simulink model "gm_spectrum_analyser"  (R2020a)
settings: Solver=VariableStepAuto  StartTime=0.0  StopTime=100000/256e6  RelTol=1e-3
InitFcn:
  | fs = 256e6;
undefined symbols (not defined in the file or in its folder): designMultirateFIR
libraries: hdlsllib x81, simulink x50, dspmlti4 x6, dsphdlxfrm x5, hdlmdlgenlib x4, dspswit3 x4, dspsigops x2, dspsigattribs x2
(part 2 of 5)

== system gm_spectrum_analyser/Stimulus and Channel/Channel/RF-DAC ==
  Valid : Inport
  Data : Inport  Port=2
  Interpolation Filter : Subsystem  mask{interp=4x}
      mask prompts: interp "Interpolation Factor:"
      mask init:
      | fir0 = dsp.FIRInterpolator('InterpolationFactor', 2,...
      |                            'CoefficientsDataType', 'Custom',...
      |                            'CustomCoefficientsDataType', numerictype([], 16, 14),...
      |                            'FullPrecisionOverride', false,...
      |                            'OutputDataType', 'Custom',...
      |                            'CustomOutputDataType', numerictype([], 16, 15),...
      |                            'Numerator', [-6, 0 54, 0, -254, 0, 1230, 2048, 1230, 0, -254, 0, 54, 0, -6]/(2048));
      | fir1 = dsp.FIRInterpolator('InterpolationFactor', 2,...
      |                            'CoefficientsDataType', 'Custom',...
      |                            'CustomCoefficientsDataType', numerictype([], 16, 14),...
      |                            'FullPrecisionOverride', false,...
      |                            'OutputDataType', 'Custom',...
      |                            'CustomOutputDataType', numerictype([], 16, 15),...
      |                            'Numerator', [-12, 0, 84, 0, -337, 0, 1008, 0, -2693, 0, 10142, 16384, 10142, 0, -2693, 0, 1008, 0, -337, 0, 84, 0 ,-12]/(16384));
      | fir2 = dsp.FIRInterpolator('InterpolationFactor', 2,...
      |                            'CoefficientsDataType', 'Custom',...
      |                            'CustomCoefficientsDataType', numerictype([], 16, 14),...
      |                            'FullPrecisionOverride', false,...
      |                            'OutputDataType', 'Custom',...
      |                            'CustomOutputDataType', numerictype([], 16, 15),...
      |                            'Numerator', [5, 0, -17, 0, 44, 0, -96, 0, 187, 0, -335, 0, 565, 0, -906, 0, 1401, 0, -2112, 0, 3145, 0, -4723, 0, 7415, 0, -13331, 0, 41526, 65536, 41526, 0, -13331, 0, 7415, 0, -4723, 0, 3145, 0, -2112, 0, 1401, 0, -906, 0, 565, 0, -335, 0, 187, 0, -96, 0, 44, 0, -17, 0, 5]/(65536));
      | switch get_param(gcb, 'interp')
      |     case '1x'
      |         if ~strcmp(get_param([gcb, '/FIR 0'], 'Commented'), 'through')
      |             set_param([gcb, '/FIR 0'],'Commented','through');
      |         end
      |         
      |         if ~strcmp(get_param([gcb, '/FIR 1'], 'Commented'), 'through')
      |             set_param([gcb, '/FIR 1'],'Commented','through');
      |         end
      |         
      |         if ~strcmp(get_param([gcb, '/FIR 2'], 'Commented'), 'through')
      |             set_param([gcb, '/FIR 2'],'Commented','through');
      |         end
      |             
      |     case '2x'
      |         if ~strcmp(get_param([gcb, '/FIR 0'], 'Commented'), 'through')
      |             set_param([gcb, '/FIR 0'],'Commented','through');
      |         end
      |         
      |         if ~strcmp(get_param([gcb, '/FIR 1'], 'Commented'), 'through')
      |             set_param([gcb, '/FIR 1'],'Commented','through');
      |         end
      |         
      |         if ~strcmp(get_param([gcb, '/FIR 2'], 'Commented'), 'off')
      |             set_param([gcb, '/FIR 2'],'Commented','off');
      |         end
      | 
      |     case '4x'
      |         if ~strcmp(get_param([gcb, '/FIR 0'], 'Commented'), 'through')
      |             set_param([gcb, '/FIR 0'],'Commented','through');
      |         end
      |         
      |         if ~strcmp(get_param([gcb, '/FIR 1'], 'Commented'), 'off')
      |             set_param([gcb, '/FIR 1'],'Commented','off');
      |         end
      |         
      |         if ~strcmp(get_param([gcb, '/FIR 2'], 'Commented'), 'off')
      |             set_param([gcb, '/FIR 2'],'Commented','off');
      |         end
      |         
      |     case '8x'
      |         if ~strcmp(get_param([gcb, '/FIR 0'], 'Commented'), 'off')
      |             set_param([gcb, '/FIR 0'],'Commented','off');
      |         end
      |         
      |         if ~strcmp(get_param([gcb, '/FIR 1'], 'Commented'), 'off')
      |             set_param([gcb, '/FIR 1'],'Commented','off');
      |         end
      |         
      |         if ~strcmp(get_param([gcb, '/FIR 2'], 'Commented'), 'off')
      |             set_param([gcb, '/FIR 2'],'Commented','off');
      |         end
      | 
      | end
      mask TypeOptions interp: 1x | 2x | 4x | 8x
      mask DialogControl DescGroupVar Prompt: RF-DAC Interpolation Filter
      mask DialogControl DescTextVar Prompt: This block simulates the RF-DAC interpolation stage using the same coefficients stored in the interpolation filters.
      mask DialogControl ParameterGroupVar Prompt: Main
  NCO and Mixer : Subsystem
  RF-DAC : Subsystem
  SSR Converter RF-DAC : Subsystem
  Data Out : Outport  VectorParamsAs1DForOutWhenUnconnected=off
  wires:
  RF-DAC/1(Data Out) -> Data Out/1
  NCO and Mixer/1(Data Out) -> RF-DAC/1(Data In)
  Interpolation Filter/1(Data Out) -> NCO and Mixer/1(Data In)
  Data/1 -> SSR Converter RF-DAC/2(Data)
  Valid/1 -> SSR Converter RF-DAC/1(Valid)
  SSR Converter RF-DAC/1(Data Out) -> Interpolation Filter/1(Data In)

== system gm_spectrum_analyser/Stimulus and Channel/Transmitter/Transmitter ==
  Enable : Inport
  Value : Inport  Port=2
  Bit Concat : hdlsllib/Logic and Bit Operations/Bit Concat  numInputs=2
  Bit Slice : hdlsllib/Logic and Bit Operations/Bit Slice  lidx=15  ridx=0
      settings: SourceProductBaseCode=SL
  Bit Slice1 : hdlsllib/Logic and Bit Operations/Bit Slice  lidx=31  ridx=16
      settings: SourceProductBaseCode=SL
  Complex to Real-Imag : ComplexToRealImag
  Constant : Constant  OutDataTypeStr=boolean  SampleTime=-1
  Constant2 : Constant  Value=[0, 0, 0, 0]'  VectorParams1D=off  OutDataTypeStr=fixdt(1,16,15)  SampleTime=-1
  Data Type Conversion : DataTypeConversion  OutDataTypeStr=fixdt(1,16,15)  ConvertRealWorld=Stored Integer (SI)
  Data Type Conversion1 : DataTypeConversion  OutDataTypeStr=fixdt(1,16,15)  ConvertRealWorld=Stored Integer (SI)
  Matrix Concatenate : Concatenate  NumInputs=4  Mode=Multidimensional array
  Multiport Switch : MultiPortSwitch  DataPortOrder=Zero-based contiguous  Inputs=2  zeroidx=on
  Real-Imag to Complex : RealImagToComplex
  Real-Imag to Complex1 : RealImagToComplex
  Vector to SSR Low : Subsystem  mask{N=4, hN=4}
      mask prompts: N "Samples per clock cycle:"
      mask init:
      | if ~isequal(get_param(gcb, 'N'), get_param(gcb, 'hN'))
      |     % Delete all blocks except input and output ports
      |     delete_block(setxor(setdiff(...
      |         find_system(gcb,'LookUnderMasks','on'),...
      |         {[gcb, '/Vector'], [gcb, '/SSR']}), gcb));
      | 
      |     % Delete all wires
      |     delete_line(find_system(gcb, 'FindAll', 'on', 'LookUnderMasks',...
      |         'on', 'SearchDepth', 3, 'Type', 'line', 'Connected', 'off'));
      | 
      |     % Add the bit concatenation block
      |     add_block('hdlsllib/Logic and Bit Operations/Bit Concat',...
      |         [gcb, '/Bit Concat'],...
      |         'Position', [155 55 205 330]);
      |     set_param([gcb, '/Bit Concat'], 'numInputs', num2str(N));
      | 
      |     % Add wire to output
      |     add_line(gcb, 'Bit Concat/1', 'SSR/1');
      | 
      |     % Add selector blocks and connect wires
      |     for i = 0:N-1
      |         add_block('simulink/Signal Routing/Selector',...
      |             [gcb, '/Selector', num2str(i)],...
      |             'Position', [0 82+i*90 45 128+i*90]);
      |         set_param([gcb, '/Selector', num2str(i)], 'InputPortWidth', num2str(N));
      |         set_param([gcb, '/Selector', num2str(i)], 'IndexParamArray', {num2str(N-i)});
      |         add_line(gcb, 'Vector/1', ['Selector', num2str(i), '/1'],...
      |             'autorouting', 'on');
      |         add_line(gcb, ['Selector', num2str(i), '/1'],...
      |             ['Bit Concat/', num2str(i+1)],...
      |             'autorouting', 'on');
      |     end
      |     
      |     % Set the hidden attribute to prevent unnecessary changes in
      |     % architecture while generating HDL Code.
      |     set_param(gcb, 'hN', get_param(gcb, 'N'));
      | end
      mask DialogControl DescGroupVar Prompt: Vector to SSR
      mask DialogControl DescTextVar Prompt: Convert a vector of inputs into SSR format.
  Valid : Outport
  Data : Outport  Port=2
  wires:
  Complex to Real-Imag/2 -> Bit Concat/1
  Vector to SSR Low/1(SSR) -> Data/1
  Complex to Real-Imag/1 -> Bit Concat/2
  Bit Concat/1 -> Vector to SSR Low/1(Vector)
  Multiport Switch/1 -> Complex to Real-Imag/1
  Constant2/1 -> Real-Imag to Complex/2, Real-Imag to Complex/1
  Real-Imag to Complex/1 -> Multiport Switch/2
  Enable/1 -> Multiport Switch/1
  Value/1 -> Bit Slice1/1, Bit Slice/1
  Data Type Conversion/1 -> Real-Imag to Complex1/1
  Bit Slice/1 -> Data Type Conversion/1
  Bit Slice1/1 -> Data Type Conversion1/1
  Data Type Conversion1/1 -> Real-Imag to Complex1/2
  Constant/1 -> Valid/1
  Real-Imag to Complex1/1 -> Matrix Concatenate/4, Matrix Concatenate/3, Matrix Concatenate/2, Matrix Concatenate/1
  Matrix Concatenate/1 -> Multiport Switch/3

== system gm_spectrum_analyser/DDR Memory/AXI Read Interface Response Model/DDR/Enabled Subsystem ==
  rd_addr : Inport
  rd_len : Inport  Port=2
  rd_avalid : Inport  Port=3
  Enable : EnablePort
  Compare To Constant : simulink/Logic and Bit Operations/Compare To Constant  relop===  const=1  OutDataTypeStr=boolean
  Constant : Constant  Value=4  SampleTime=-1
  Constant1 : Constant  OutDataTypeStr=boolean  SampleTime=-1
  Delay : Delay  DelayLength=1
  Direct Lookup Table (n-D) : LookupNDDirect  NumberOfTableDimensions=1  Table=DDR_DATA  DiagnosticForOutOfRangeInput=Error
  HDL Counter : hdlsllib/Sources/HDL Counter  CountType=Count limited  CountInit=0  CountStep=1  CountMax=2^16-1  CountFromType=Specify  CountFrom=0  CountResetPort=on  CountLoadPort=off  CountEnbPort=on  CountDirPort=off  CountDataType=Unsigned  CountWordLen=16  CountFracLen=0  CountSampTime=1
  MATLAB Function : MATLAB Function  TreatAsAtomicUnit=on
  Product : Product  Inputs=*/
  Sum : Sum  Inputs=|++  OutDataTypeStr=uint32
  Sum1 : Sum  Inputs=|+-
  latch : Subsystem
  rd_data : Outport  VectorParamsAs1DForOutWhenUnconnected=off
  rd_aready : Outport  Port=2  VectorParamsAs1DForOutWhenUnconnected=off
  rd_dvalid : Outport  Port=3  VectorParamsAs1DForOutWhenUnconnected=off
  wires:
  Constant1/1 -> rd_aready/1
  Delay/1 -> MATLAB Function/2(rst)
  Constant/1 -> Product/2
  Product/1 -> Sum/1
  latch/1(q) -> Product/1
  MATLAB Function/1(start_counter) -> HDL Counter/2, rd_dvalid/1
  rd_avalid/1 -> MATLAB Function/1(rd_avalid), latch/1(e)
  rd_len/1 -> Sum1/1
  rd_addr/1 -> latch/2(d)
  Compare To Constant/1 -> HDL Counter/1, Delay/1
  Sum/1 -> Direct Lookup Table (n-D)/1
  Sum1/1 -> Compare To Constant/1
  HDL Counter/1 -> Sum/2, Sum1/2  "addr_inc"
  Direct Lookup Table (n-D)/1 -> rd_data/1

== system gm_spectrum_analyser/DDR Memory/AXI Write Interface Response Model/Serial to FFT Frame/Enabled Subsystem2 ==
  Data In : Inport
  Enable : EnablePort
  Buffer : Buffer  N=N  OutputFrames=off
  Data Out : Outport
  wires:
  Data In/1 -> Buffer/1
  Buffer/1 -> Data Out/1

== system gm_spectrum_analyser/Spectrum Analyser/Spectrum Analyser/Direct Memory Access/Direct Memory Access ==
  Length : Inport  OutDataTypeStr=uint32  PortDimensions=1  SampleTime=3.90625e-09
  Count : Inport  Port=2  OutDataTypeStr=uint32  PortDimensions=1  SampleTime=3.90625e-09
  Buffer Address 1 : Inport  Port=3  OutDataTypeStr=uint32  PortDimensions=1  SampleTime=3.90625e-09
  Buffer Address 2 : Inport  Port=4  OutDataTypeStr=uint32  PortDimensions=1  SampleTime=3.90625e-09
  Buffer Address 3 : Inport  Port=5  OutDataTypeStr=uint32  PortDimensions=1  SampleTime=3.90625e-09
  Enable DMA : Inport  Port=6  OutDataTypeStr=uint32  PortDimensions=1  SampleTime=3.90625e-09
  Valid In : Inport  Port=7  OutDataTypeStr=boolean  PortDimensions=1  SampleTime=3.90625e-09
  Data In : Inport  Port=8  OutDataTypeStr=uint32  PortDimensions=1  SampleTime=3.90625e-09
  Start In : Inport  Port=9  OutDataTypeStr=boolean  PortDimensions=1  SampleTime=3.90625e-09
  End In : Inport  Port=10  OutDataTypeStr=boolean  PortDimensions=1  SampleTime=3.90625e-09
  wr_ready : Inport  Port=11  SampleTime=3.90625e-09
  DDR Communication : Subsystem
  wr_data : Outport
  wr_m2s : Outport  Port=2
  Buffer Pointer : Outport  Port=3
  DMA Status : Outport  Port=4
  wires:
  DDR Communication/1(Buffer Pointer) -> Buffer Pointer/1
  DDR Communication/2(wr_data) -> wr_data/1
  DDR Communication/3(wr_m2s) -> wr_m2s/1
  DDR Communication/4(DMA Status) -> DMA Status/1
  Length/1 -> DDR Communication/1(Length)
  Count/1 -> DDR Communication/2(Count)
  Buffer Address 1/1 -> DDR Communication/3(Buffer Address 1)
  Buffer Address 2/1 -> DDR Communication/4(Buffer Address 2)
  Buffer Address 3/1 -> DDR Communication/5(Buffer Address 3)
  Enable DMA/1 -> DDR Communication/6(Enable)
  Valid In/1 -> DDR Communication/7(Valid Out)
  Data In/1 -> DDR Communication/8(Data Out)
  Start In/1 -> DDR Communication/9(Start In)
  End In/1 -> DDR Communication/10(End In)
  wr_ready/1 -> DDR Communication/11(wr_ready)

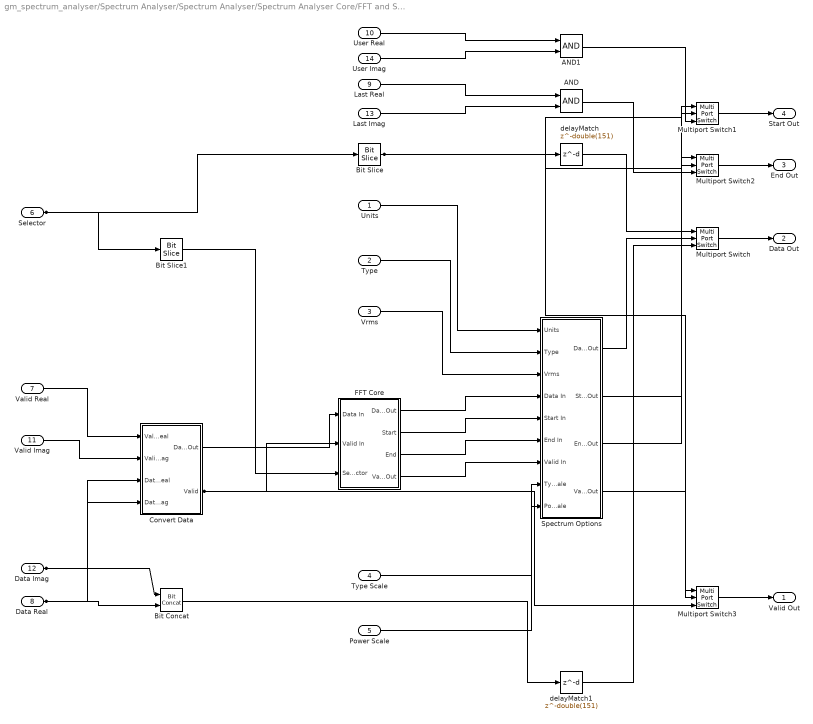
== system gm_spectrum_analyser/Spectrum Analyser/Spectrum Analyser/Spectrum Analyser Core/FFT and Spectrum Processing ==
  Units : Inport  OutDataTypeStr=uint32  SampleTime=3.90625e-09
  Type : Inport  Port=2  OutDataTypeStr=uint32  SampleTime=3.90625e-09
  Vrms : Inport  Port=3  OutDataTypeStr=uint32  SampleTime=3.90625e-09
  Type Scale : Inport  Port=4  OutDataTypeStr=uint32  SampleTime=3.90625e-09
  Power Scale : Inport  Port=5  OutDataTypeStr=uint32  SampleTime=3.90625e-09
  Selector : Inport  Port=6  OutDataTypeStr=uint32  SampleTime=3.90625e-09
  Valid Real : Inport  Port=7  OutDataTypeStr=boolean  SampleTime=3.90625e-09
  Data Real : Inport  Port=8  OutDataTypeStr=uint16  SampleTime=3.90625e-09
  Last Real : Inport  Port=9  OutDataTypeStr=boolean  SampleTime=3.90625e-09
  User Real : Inport  Port=10  OutDataTypeStr=boolean  SampleTime=3.90625e-09
  Valid Imag : Inport  Port=11  OutDataTypeStr=boolean  SampleTime=3.90625e-09
  Data Imag : Inport  Port=12  OutDataTypeStr=uint16  SampleTime=3.90625e-09
  Last Imag : Inport  Port=13  OutDataTypeStr=boolean  SampleTime=3.90625e-09
  User Imag : Inport  Port=14  OutDataTypeStr=boolean  SampleTime=3.90625e-09
  AND : Logic  AllPortsSameDT=off  OutDataTypeStr=boolean  SampleTime=3.90625e-09
  AND1 : Logic  AllPortsSameDT=off  OutDataTypeStr=boolean  SampleTime=3.90625e-09
  Bit Concat : hdlsllib/Logic and Bit Operations/Bit Concat  numInputs=2
  Bit Slice : hdlsllib/Logic and Bit Operations/Bit Slice  lidx=double(8)  ridx=double(8)
      settings: SourceProductBaseCode=SL
  Bit Slice1 : hdlsllib/Logic and Bit Operations/Bit Slice  lidx=double(7)  ridx=double(0)
      settings: SourceProductBaseCode=SL
  Convert Data : Subsystem
  FFT Core : Subsystem
  Multiport Switch : MultiPortSwitch  DataPortOrder=Zero-based contiguous  Inputs=2  DiagnosticForDefault=None  zeroidx=on  OutDataTypeStr=uint32  SampleTime=3.90625e-09
  Multiport Switch1 : MultiPortSwitch  DataPortOrder=Zero-based contiguous  Inputs=2  DiagnosticForDefault=None  zeroidx=on  SampleTime=3.90625e-09
  Multiport Switch2 : MultiPortSwitch  DataPortOrder=Zero-based contiguous  Inputs=2  DiagnosticForDefault=None  zeroidx=on  SampleTime=3.90625e-09
  Multiport Switch3 : MultiPortSwitch  DataPortOrder=Zero-based contiguous  Inputs=2  DiagnosticForDefault=None  zeroidx=on  SampleTime=3.90625e-09
  Spectrum Options : Subsystem
  delayMatch : Delay  DelayLength=double(151)  InitialCondition=0  SampleTime=3.90625e-09
  delayMatch1 : Delay  DelayLength=double(151)  InitialCondition=0  SampleTime=3.90625e-09
  Valid Out : Outport
  Data Out : Outport  Port=2
  End Out : Outport  Port=3
  Start Out : Outport  Port=4
  wires:
  AND/1 -> Multiport Switch2/3
  AND1/1 -> Multiport Switch1/3
  delayMatch1/1 -> Multiport Switch/3
  delayMatch/1 -> Multiport Switch/1
  Bit Slice1/1 -> FFT Core/3(Selector)
  Convert Data/1(Data Out) -> FFT Core/1(Data In)
  Convert Data/2(Valid) -> Multiport Switch3/3, FFT Core/2(Valid In)
  FFT Core/1(Data Out) -> Spectrum Options/4(Data In)
  FFT Core/2(Start) -> Spectrum Options/5(Start In)
  FFT Core/3(End) -> Spectrum Options/6(End In)
  FFT Core/4(Valid Out) -> Spectrum Options/7(Valid In)
  Multiport Switch/1 -> Data Out/1
  Multiport Switch1/1 -> Start Out/1
  Multiport Switch2/1 -> End Out/1
  Multiport Switch3/1 -> Valid Out/1
  Spectrum Options/1(Data Out) -> Multiport Switch/2
  Spectrum Options/2(Start Out) -> Multiport Switch1/2
  Spectrum Options/3(End Out) -> Multiport Switch2/2
  Spectrum Options/4(Valid Out) -> Multiport Switch3/2
  Bit Slice/1 -> delayMatch/1, Multiport Switch3/1, Multiport Switch2/1, Multiport Switch1/1
  Bit Concat/1 -> delayMatch1/1
  Units/1 -> Spectrum Options/1(Units)
  Type/1 -> Spectrum Options/2(Type)
  Vrms/1 -> Spectrum Options/3(Vrms)
  Type Scale/1 -> Spectrum Options/8(Type Scale)
  Power Scale/1 -> Spectrum Options/9(Power Scale)
  Selector/1 -> Bit Slice1/1, Bit Slice/1
  Valid Real/1 -> Convert Data/1(Valid Real)
  Data Real/1 -> Bit Concat/2, Convert Data/3(Data Real)
  Last Real/1 -> AND/1
  User Real/1 -> AND1/1
  Valid Imag/1 -> Convert Data/2(Valid Imag)
  Data Imag/1 -> Bit Concat/1, Convert Data/4(Data Imag)
  Last Imag/1 -> AND/2
  User Imag/1 -> AND1/2

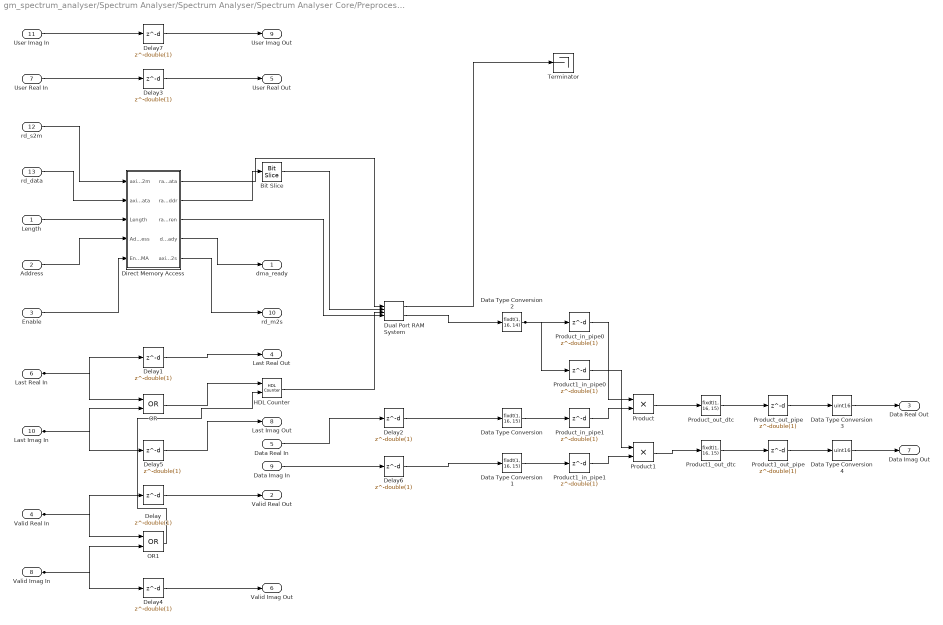
== system gm_spectrum_analyser/Spectrum Analyser/Spectrum Analyser/Spectrum Analyser Core/Preprocessing Window ==
  Length : Inport  OutDataTypeStr=uint32  SampleTime=3.90625e-09
  Address : Inport  Port=2  OutDataTypeStr=uint32  SampleTime=3.90625e-09
  Enable : Inport  Port=3  OutDataTypeStr=uint32  SampleTime=3.90625e-09
  Valid Real In : Inport  Port=4  OutDataTypeStr=boolean  SampleTime=3.90625e-09
  Data Real In : Inport  Port=5  OutDataTypeStr=uint16  SampleTime=3.90625e-09
  Last Real In : Inport  Port=6  OutDataTypeStr=boolean  SampleTime=3.90625e-09
  User Real In : Inport  Port=7  OutDataTypeStr=boolean  SampleTime=3.90625e-09
  Valid Imag In : Inport  Port=8  OutDataTypeStr=boolean  SampleTime=3.90625e-09
  Data Imag In : Inport  Port=9  OutDataTypeStr=uint16  SampleTime=3.90625e-09
  Last Imag In : Inport  Port=10  OutDataTypeStr=boolean  SampleTime=3.90625e-09
  User Imag In : Inport  Port=11  OutDataTypeStr=boolean  SampleTime=3.90625e-09
  rd_s2m : Inport  Port=12  SampleTime=3.90625e-09
  rd_data : Inport  Port=13  OutDataTypeStr=uint16  SampleTime=3.90625e-09
  Bit Slice : hdlsllib/Logic and Bit Operations/Bit Slice  lidx=double(12)  ridx=double(0)
      settings: SourceProductBaseCode=SL
  Data Type Conversion : DataTypeConversion  OutDataTypeStr=fixdt(1, 16, 15)  ConvertRealWorld=Stored Integer (SI)  SampleTime=3.90625e-09
  Data Type Conversion1 : DataTypeConversion  OutDataTypeStr=fixdt(1, 16, 15)  ConvertRealWorld=Stored Integer (SI)  SampleTime=3.90625e-09
  Data Type Conversion2 : DataTypeConversion  OutDataTypeStr=fixdt(1, 16, 14)  ConvertRealWorld=Stored Integer (SI)  SampleTime=3.90625e-09
  Data Type Conversion3 : DataTypeConversion  OutDataTypeStr=uint16  ConvertRealWorld=Stored Integer (SI)  SampleTime=3.90625e-09
  Data Type Conversion4 : DataTypeConversion  OutDataTypeStr=uint16  ConvertRealWorld=Stored Integer (SI)  SampleTime=3.90625e-09
  Delay{,1..7} (8 alike) : Delay  DelayLength=double(1)  InitialCondition=0  SampleTime=3.90625e-09
  Direct Memory Access : Subsystem
  Dual Port RAM System : hdlsllib/HDL RAMs/Dual Port RAM System  RAMType=Dual port  WriteOutputValue=New data  RAMInitialValue=ones(1, 2^13)*2^14  SimulateUsing=Code generation
      settings: SourceProductBaseCode=SL
  HDL Counter : hdlsllib/Sources/HDL Counter  CountType=Count limited  CountInit=double(0)  CountStep=double(1)  CountMax=double(8191)  CountFromType=Initial value  CountFrom=double(0)  CountResetPort=on  CountLoadPort=off  CountEnbPort=on  CountDirPort=off  CountDataType=Unsigned  CountWordLen=13  CountFracLen=0  CountSampTime=3.90625e-09
  OR : Logic  Operator=OR  AllPortsSameDT=off  OutDataTypeStr=boolean  SampleTime=3.90625e-09
  OR1 : Logic  Operator=OR  AllPortsSameDT=off  OutDataTypeStr=boolean  SampleTime=3.90625e-09
  Product : Product  Inputs=**  OutDataTypeStr=fixdt(1, 32, 29)  SampleTime=3.90625e-09
  Product1 : Product  Inputs=**  OutDataTypeStr=fixdt(1, 32, 29)  SampleTime=3.90625e-09
  Product1_in_pipe0 : Delay  DelayLength=double(1)  InitialCondition=0  SampleTime=3.90625e-09
  Product1_in_pipe1 : Delay  DelayLength=double(1)  InitialCondition=0  SampleTime=3.90625e-09
  Product1_out_dtc : DataTypeConversion  OutDataTypeStr=fixdt(1, 16, 15)  RndMeth=Round  SampleTime=3.90625e-09  SaturateOnIntegerOverflow=on
  Product1_out_pipe : Delay  DelayLength=double(1)  InitialCondition=0  SampleTime=3.90625e-09
  Product_in_pipe0 : Delay  DelayLength=double(1)  InitialCondition=0  SampleTime=3.90625e-09
  Product_in_pipe1 : Delay  DelayLength=double(1)  InitialCondition=0  SampleTime=3.90625e-09
  Product_out_dtc : DataTypeConversion  OutDataTypeStr=fixdt(1, 16, 15)  RndMeth=Round  SampleTime=3.90625e-09  SaturateOnIntegerOverflow=on
  Product_out_pipe : Delay  DelayLength=double(1)  InitialCondition=0  SampleTime=3.90625e-09
  Terminator : Terminator
  dma_ready : Outport
  Valid Real Out : Outport  Port=2
  Data Real Out : Outport  Port=3
  Last Real Out : Outport  Port=4
  User Real Out : Outport  Port=5
  Valid Imag Out : Outport  Port=6
  Data Imag Out : Outport  Port=7
  Last Imag Out : Outport  Port=8
  User Imag Out : Outport  Port=9
  rd_m2s : Outport  Port=10
  wires:
  Bit Slice/1 -> Dual Port RAM System/2
  Data Type Conversion/1 -> Product_in_pipe1/1
  Data Type Conversion1/1 -> Product1_in_pipe1/1
  Data Type Conversion2/1 -> Product1_in_pipe0/1, Product_in_pipe0/1
  Data Type Conversion3/1 -> Data Real Out/1
  Data Type Conversion4/1 -> Data Imag Out/1
  Delay/1 -> Valid Real Out/1
  Delay1/1 -> Last Real Out/1
  Delay2/1 -> Data Type Conversion/1
  Delay3/1 -> User Real Out/1
  Delay4/1 -> Valid Imag Out/1
  Delay5/1 -> Last Imag Out/1
  Delay6/1 -> Data Type Conversion1/1
  Delay7/1 -> User Imag Out/1
  Direct Memory Access/1(ram_wr_data) -> Dual Port RAM System/1
  Direct Memory Access/2(ram_wr_addr) -> Bit Slice/1
  Direct Memory Access/3(ram_wren) -> Dual Port RAM System/3
  Direct Memory Access/4(dma_read_ready) -> dma_ready/1
  Direct Memory Access/5(axim_rd_m2s) -> rd_m2s/1
  Dual Port RAM System/1 -> Terminator/1
  Dual Port RAM System/2 -> Data Type Conversion2/1
  HDL Counter/1 -> Dual Port RAM System/4
  OR/1 -> HDL Counter/1
  OR1/1 -> HDL Counter/2
  Product_out_pipe/1 -> Data Type Conversion3/1
  Product1_out_pipe/1 -> Data Type Conversion4/1
  Product_out_dtc/1 -> Product_out_pipe/1
  Product1_out_dtc/1 -> Product1_out_pipe/1
  Product_in_pipe0/1 -> Product/1
  Product_in_pipe1/1 -> Product/2
  Product1_in_pipe0/1 -> Product1/1
  Product1_in_pipe1/1 -> Product1/2
  Product/1 -> Product_out_dtc/1
  Product1/1 -> Product1_out_dtc/1
  Length/1 -> Direct Memory Access/3(Length)
  Address/1 -> Direct Memory Access/4(Address)
  Enable/1 -> Direct Memory Access/5(Enable DMA)
  Valid Real In/1 -> OR1/1, Delay/1
  Data Real In/1 -> Delay2/1
  Last Real In/1 -> OR/1, Delay1/1
  User Real In/1 -> Delay3/1
  Valid Imag In/1 -> OR1/2, Delay4/1
  Data Imag In/1 -> Delay6/1
  Last Imag In/1 -> OR/2, Delay5/1
  User Imag In/1 -> Delay7/1
  rd_s2m/1 -> Direct Memory Access/1(axim_rd_s2m)
  rd_data/1 -> Direct Memory Access/2(axim_rd_data)

== system gm_spectrum_analyser/Spectrum Analyser/Spectrum Analyser/Spectrum Analyser Core/SSR Subset Converter ==
  Packet Size : Inport  OutDataTypeStr=uint32  SampleTime=3.90625e-09
  SSR Mode : Inport  Port=2  OutDataTypeStr=uint32  SampleTime=3.90625e-09
  Valid Real In : Inport  Port=3  OutDataTypeStr=boolean  SampleTime=3.90625e-09
  Data Real In : Inport  Port=4  OutDataTypeStr=fixdt(0, 128, 0)  SampleTime=3.90625e-09
  Valid Imag In : Inport  Port=5  OutDataTypeStr=boolean  SampleTime=3.90625e-09
  Data Imag In : Inport  Port=6  OutDataTypeStr=fixdt(0, 128, 0)  SampleTime=3.90625e-09
  Bit Slice : hdlsllib/Logic and Bit Operations/Bit Slice  lidx=double(3)  ridx=double(0)
      settings: SourceProductBaseCode=SL
  SSR Deserializer Imag : Subsystem
  SSR Deserializer Real : Subsystem
  SSR Packet Generator Imag : Subsystem
  SSR Packet Generator Real : Subsystem
  SSR Serializer Imag : Subsystem
  SSR Serializer Real : Subsystem
  Valid Real Out : Outport
  Data Real Out : Outport  Port=2
  Last Real Out : Outport  Port=3
  User Real Out : Outport  Port=4
  Valid Imag Out : Outport  Port=5
  Data Imag Out : Outport  Port=6
  Last Imag Out : Outport  Port=7
  User Imag Out : Outport  Port=8
  wires:
  Bit Slice/1 -> SSR Packet Generator Imag/1(Frame Drop), SSR Packet Generator Real/1(Frame Drop), SSR Serializer Imag/1(SSR Control), SSR Serializer Real/1(SSR Control)
  SSR Deserializer Imag/1(Valid Out) -> Valid Imag Out/1
  SSR Deserializer Imag/2(Data Out) -> Data Imag Out/1
  SSR Deserializer Imag/3(SoF Out) -> User Imag Out/1
  SSR Deserializer Imag/4(EoL Out) -> Last Imag Out/1
  SSR Deserializer Real/1(Valid Out) -> Valid Real Out/1
  SSR Deserializer Real/2(Data Out) -> Data Real Out/1
  SSR Deserializer Real/3(SoF Out) -> User Real Out/1
  SSR Deserializer Real/4(EoL Out) -> Last Real Out/1
  SSR Packet Generator Imag/1(Valid Out) -> SSR Deserializer Imag/1(Valid In)
  SSR Packet Generator Imag/2(Data Out) -> SSR Deserializer Imag/2(Data In)
  SSR Packet Generator Imag/3(SoF Out) -> SSR Deserializer Imag/3(SoF In)
  SSR Packet Generator Imag/4(EoF Out) -> SSR Deserializer Imag/4(EoF In)
  SSR Packet Generator Real/1(Valid Out) -> SSR Deserializer Real/1(Valid In)
  SSR Packet Generator Real/2(Data Out) -> SSR Deserializer Real/2(Data In)
  SSR Packet Generator Real/3(SoF Out) -> SSR Deserializer Real/3(SoF In)
  SSR Packet Generator Real/4(EoF Out) -> SSR Deserializer Real/4(EoF In)
  SSR Serializer Imag/1(Valid Out) -> SSR Packet Generator Imag/2(Valid In)
  SSR Serializer Imag/2(Data Out) -> SSR Packet Generator Imag/3(Data In)
  SSR Serializer Real/1(Valid Out) -> SSR Packet Generator Real/2(Valid In)
  SSR Serializer Real/2(Data Out) -> SSR Packet Generator Real/3(Data In)
  Packet Size/1 -> SSR Packet Generator Imag/4(Packet Size), SSR Packet Generator Real/4(Packet Size)
  SSR Mode/1 -> Bit Slice/1
  Valid Real In/1 -> SSR Serializer Real/2(Valid In)
  Data Real In/1 -> SSR Serializer Real/3(Data In)
  Valid Imag In/1 -> SSR Serializer Imag/2(Valid In)
  Data Imag In/1 -> SSR Serializer Imag/3(Data In)

== system gm_spectrum_analyser/Stimulus and Channel/Channel/RF-ADC/Decimation Filter ==
  Data In : Inport
  FIR 0 : dspmlti4/FIR Decimation  FilterSource=Filter object  h=designMultirateFIR(1,2)  D=2  filtStruct=Direct form  FilterObject=fir0  InputProcessing=Columns as channels (frame based)  framing=Allow multirate processing  inputOffset=0  outputBufInitCond=0  roundingMode=Floor  overflowMode=off  firstCoeffDataTypeStr=Inherit: Same word length as input  firstCoeffMin=[]  firstCoeffMax=[]  firstCoeffLastDataTypeStr=Inherit: Same word length as input  outputDataTypeStr=Inherit: Same as accumulator  outputMin=[]  outputMax=[]  outputLastDataTypeStr=Inherit: Same as accumulator
  FIR 1 : dspmlti4/FIR Decimation  Commented=through  FilterSource=Filter object  h=designMultirateFIR(1,2)  D=2  filtStruct=Direct form  FilterObject=fir1  InputProcessing=Columns as channels (frame based)  framing=Allow multirate processing  inputOffset=0  outputBufInitCond=0  roundingMode=Floor  overflowMode=off  firstCoeffDataTypeStr=Inherit: Same word length as input  firstCoeffMin=[]  firstCoeffMax=[]  firstCoeffLastDataTypeStr=Inherit: Same word length as input  outputDataTypeStr=Inherit: Same as accumulator  outputMin=[]  outputMax=[]  outputLastDataTypeStr=Inherit: Same as accumulator
  FIR 2 : dspmlti4/FIR Decimation  Commented=through  FilterSource=Filter object  h=designMultirateFIR(1,2)  D=2  filtStruct=Direct form  FilterObject=fir2  InputProcessing=Columns as channels (frame based)  framing=Allow multirate processing  inputOffset=0  outputBufInitCond=0  roundingMode=Floor  overflowMode=off  firstCoeffDataTypeStr=Inherit: Same word length as input  firstCoeffMin=[]  firstCoeffMax=[]  firstCoeffLastDataTypeStr=Inherit: Same word length as input  outputDataTypeStr=Inherit: Same as accumulator  outputMin=[]  outputMax=[]  outputLastDataTypeStr=Inherit: Same as accumulator
  Data Out : Outport  VectorParamsAs1DForOutWhenUnconnected=off
  wires:
  FIR 2/1 -> Data Out/1
  Data In/1 -> FIR 0/1
  FIR 0/1 -> FIR 1/1
  FIR 1/1 -> FIR 2/1

== system gm_spectrum_analyser/Stimulus and Channel/Channel/RF-ADC/NCO and Mixer ==
  Data In : Inport
  Constant1 : Constant  Value=m  OutDataTypeStr=fixdt(0,2,0)  SampleTime=-1
  Data Type Conversion : DataTypeConversion  OutDataTypeStr=fixdt(1,16,15)
  Multiport Switch1 : MultiPortSwitch  DataPortOrder=Zero-based contiguous  zeroidx=on
  RF-ADC Coarse Mixer : Subsystem
  RF-ADC Fine Mixer : Subsystem
  Real-Imag to Complex : RealImagToComplex
  Data Out : Outport  VectorParamsAs1DForOutWhenUnconnected=off
  wires:
  Multiport Switch1/1 -> Data Out/1
  RF-ADC Fine Mixer/1(Data Out) -> Multiport Switch1/4
  Real-Imag to Complex/1 -> Data Type Conversion/1
  RF-ADC Coarse Mixer/1(Data Out) -> Multiport Switch1/3
  Data In/1 -> Real-Imag to Complex/1, RF-ADC Coarse Mixer/1(Data In), RF-ADC Fine Mixer/1(Data In), Real-Imag to Complex/2
  Constant1/1 -> Multiport Switch1/1
  Data Type Conversion/1 -> Multiport Switch1/2

== system gm_spectrum_analyser/Stimulus and Channel/Channel/RF-ADC/RF-ADC ==
  Data In : Inport
  Buffer : Buffer  N=ssr  OutputFrames=off
  Data Type Conversion : DataTypeConversion  OutDataTypeStr=fixdt(1,12,11)  SaturateOnIntegerOverflow=on
  Rate Transition : RateTransition  OutPortSampleTime=1/fs
  Data Out : Outport  VectorParamsAs1DForOutWhenUnconnected=off
  wires:
  Rate Transition/1 -> Data Type Conversion/1
  Data In/1 -> Rate Transition/1
  Data Type Conversion/1 -> Buffer/1
  Buffer/1 -> Data Out/1

== system gm_spectrum_analyser/Stimulus and Channel/Channel/RF-ADC/SSR Converter RF-ADC ==
  Real In : Inport
  Imag In : Inport  Port=2
  Constant : Constant  OutDataTypeStr=boolean  SampleTime=-1
  Convert 2-D to 1-D : dspsigattribs/Convert 2-D to 1-D
      settings: SourceProductBaseCode=DS
  Convert 2-D to 1-D1 : dspsigattribs/Convert 2-D to 1-D
      settings: SourceProductBaseCode=DS
  Vector to SSR Imag : Subsystem  mask{N=8, hN=8}
      mask prompts: N "Samples per clock cycle:"
      mask init:
      | if ~isequal(get_param(gcb, 'N'), get_param(gcb, 'hN'))
      |     % Delete all blocks except input and output ports
      |     delete_block(setxor(setdiff(...
      |         find_system(gcb,'LookUnderMasks','on'),...
      |         {[gcb, '/Vector'], [gcb, '/SSR']}), gcb));
      | 
      |     % Delete all wires
      |     delete_line(find_system(gcb, 'FindAll', 'on', 'LookUnderMasks',...
      |         'on', 'SearchDepth', 3, 'Type', 'line', 'Connected', 'off'));
      | 
      |     % Add the bit concatenation block
      |     add_block('hdlsllib/Logic and Bit Operations/Bit Concat',...
      |         [gcb, '/Bit Concat'],...
      |         'Position', [155 55 205 330]);
      |     set_param([gcb, '/Bit Concat'], 'numInputs', num2str(N));
      | 
      |     % Add wire to output
      |     add_line(gcb, 'Bit Concat/1', 'SSR/1');
      | 
      |     % Add selector blocks and connect wires
      |     for i = 0:N-1
      |         add_block('simulink/Signal Routing/Selector',...
      |             [gcb, '/Selector', num2str(i)],...
      |             'Position', [0 82+i*90 45 128+i*90]);
      |         set_param([gcb, '/Selector', num2str(i)], 'InputPortWidth', num2str(N), 'IndexParamArray', {num2str(N-i)});
      |         add_line(gcb, 'Vector/1', ['Selector', num2str(i), '/1'],...
      |             'autorouting', 'on');
      |         add_line(gcb, ['Selector', num2str(i), '/1'],...
      |             ['Bit Concat/', num2str(i+1)],...
      |             'autorouting', 'on');
      |     end
      |     
      |     % Set the hidden attribute to prevent unnecessary changes in
      |     % architecture while generating HDL Code.
      |     set_param(gcb, 'hN', get_param(gcb, 'N'));
      | end
      mask DialogControl DescGroupVar Prompt: Vector to SSR
      mask DialogControl DescTextVar Prompt: Convert a vector of inputs into SSR format.
  Vector to SSR Real : Subsystem  mask{N=8, hN=8}
      mask prompts: N "Samples per clock cycle:"
      mask init: same as gm_spectrum_analyser/Stimulus and Channel/Channel/RF-ADC/SSR Converter RF-ADC/Vector to SSR Imag
      mask DialogControl DescGroupVar Prompt: Vector to SSR
      mask DialogControl DescTextVar Prompt: Convert a vector of inputs into SSR format.
  Valid Real : Outport
  Valid Imag : Outport  Port=2
  Real Out : Outport  Port=3
  Imag Out : Outport  Port=4
  wires:
  Real In/1 -> Convert 2-D to 1-D/1
  Imag In/1 -> Convert 2-D to 1-D1/1
  Convert 2-D to 1-D/1 -> Vector to SSR Real/1(Vector)
  Convert 2-D to 1-D1/1 -> Vector to SSR Imag/1(Vector)
  Vector to SSR Real/1(SSR) -> Real Out/1
  Vector to SSR Imag/1(SSR) -> Imag Out/1
  Constant/1 -> Valid Imag/1, Valid Real/1

== system gm_spectrum_analyser/Stimulus and Channel/Channel/RF-DAC/Interpolation Filter ==
  Data In : Inport
  FIR 0 : dspmlti4/FIR Interpolation  Commented=through  FilterSource=Filter object  PrivateCoeffs=0  h=designMultirateFIR(3,1)  L=2  FilterObject=fir0  InputProcessing=Columns as channels (frame based)  framing=Allow multirate processing  outputBufInitCond=0  roundingMode=Floor  overflowMode=off  firstCoeffDataTypeStr=Inherit: Same word length as input  firstCoeffMin=[]  firstCoeffMax=[]  firstCoeffLastDataTypeStr=Inherit: Same word length as input  outputDataTypeStr=Inherit: Same as accumulator  outputMin=[]  outputMax=[]  outputLastDataTypeStr=Inherit: Same as accumulator
  FIR 1 : dspmlti4/FIR Interpolation  FilterSource=Filter object  PrivateCoeffs=0  h=designMultirateFIR(3,1)  L=2  FilterObject=fir1  InputProcessing=Columns as channels (frame based)  framing=Allow multirate processing  outputBufInitCond=0  roundingMode=Floor  overflowMode=off  firstCoeffDataTypeStr=Inherit: Same word length as input  firstCoeffMin=[]  firstCoeffMax=[]  firstCoeffLastDataTypeStr=Inherit: Same word length as input  outputDataTypeStr=Inherit: Same as accumulator  outputMin=[]  outputMax=[]  outputLastDataTypeStr=Inherit: Same as accumulator
  FIR 2 : dspmlti4/FIR Interpolation  FilterSource=Filter object  PrivateCoeffs=0  h=designMultirateFIR(3,1)  L=2  FilterObject=fir2  InputProcessing=Columns as channels (frame based)  framing=Allow multirate processing  outputBufInitCond=0  roundingMode=Floor  overflowMode=off  firstCoeffDataTypeStr=Inherit: Same word length as input  firstCoeffMin=[]  firstCoeffMax=[]  firstCoeffLastDataTypeStr=Inherit: Same word length as input  outputDataTypeStr=Inherit: Same as accumulator  outputMin=[]  outputMax=[]  outputLastDataTypeStr=Inherit: Same as accumulator
  Data Out : Outport  VectorParamsAs1DForOutWhenUnconnected=off
  wires:
  FIR 2/1 -> FIR 1/1
  Data In/1 -> FIR 2/1
  FIR 0/1 -> Data Out/1
  FIR 1/1 -> FIR 0/1

== system gm_spectrum_analyser/Stimulus and Channel/Channel/RF-DAC/NCO and Mixer ==
  Data In : Inport
  Complex to Real-Imag : ComplexToRealImag
  Constant1 : Constant  Value=m  OutDataTypeStr=fixdt(0,2,0)  SampleTime=-1
  Multiport Switch1 : MultiPortSwitch  DataPortOrder=Zero-based contiguous  zeroidx=on
  RF-DAC Coarse Mixer : Subsystem
  RF-DAC Fine Mixer : Subsystem
  Terminator : Terminator
  Data Out : Outport  VectorParamsAs1DForOutWhenUnconnected=off
  wires:
  RF-DAC Coarse Mixer/1(Data Out) -> Multiport Switch1/3
  Constant1/1 -> Multiport Switch1/1
  Data In/1 -> Complex to Real-Imag/1, RF-DAC Coarse Mixer/1(Data In), RF-DAC Fine Mixer/1(Data In)
  Multiport Switch1/1 -> Data Out/1
  RF-DAC Fine Mixer/1(Data Out) -> Multiport Switch1/4
  Complex to Real-Imag/1 -> Multiport Switch1/2
  Complex to Real-Imag/2 -> Terminator/1

== system gm_spectrum_analyser/Stimulus and Channel/Channel/RF-DAC/RF-DAC ==
  Data In : Inport
  Cast To Double : DataTypeConversion  OutDataTypeStr=double
  Rate Transition : RateTransition  OutPortSampleTime=0
  Unbuffer : Unbuffer
  Data Out : Outport  VectorParamsAs1DForOutWhenUnconnected=off
  wires:
  Cast To Double/1 -> Rate Transition/1
  Unbuffer/1 -> Cast To Double/1
  Data In/1 -> Unbuffer/1
  Rate Transition/1 -> Data Out/1

== system gm_spectrum_analyser/Stimulus and Channel/Channel/RF-DAC/SSR Converter RF-DAC ==
  Valid : Inport
  Data : Inport  Port=2
  Bit Slice Imag1 : hdlsllib/Logic and Bit Operations/Bit Slice  lidx=31  ridx=16
      settings: SourceProductBaseCode=SL
  Bit Slice Real1 : hdlsllib/Logic and Bit Operations/Bit Slice  lidx=15  ridx=0
      settings: SourceProductBaseCode=SL
  Data Type Conversion : DataTypeConversion  OutDataTypeStr=fixdt(1,16,15)  ConvertRealWorld=Stored Integer (SI)
  Real-Imag to Complex1 : RealImagToComplex
  SSR to Vector Low : Subsystem  mask{N=ssr, w=32, hN=ssr, hw=32}
      mask prompts: N "Samples per clock cycle:"; w "Wordlength:"
      mask init:
      | if ~isequal(get_param(gcb, 'N'), get_param(gcb, 'hN')) ||...
      |         ~isequal(get_param(gcb, 'w'), get_param(gcb, 'hw'))
      |     % Delete all blocks except input and output ports
      |     delete_block(setxor(setdiff(...
      |         find_system(gcb,'LookUnderMasks','on'),...
      |         {[gcb, '/Vector'], [gcb, '/SSR']}), gcb));
      | 
      |     % Delete all wires
      |     delete_line(find_system(gcb, 'FindAll', 'on', 'LookUnderMasks',...
      |         'on', 'SearchDepth', 3, 'Type', 'line', 'Connected', 'off'));
      | 
      |     % Add the matrix concatenation block
      |     add_block('hdlsllib/Math Operations/Matrix Concatenate',...
      |         [gcb, '/Matrix Concatenate'],...
      |         'Position', [155 55 205 330]);
      |     set_param([gcb, '/Matrix Concatenate'], 'NumInputs', num2str(N));
      |     set_param([gcb, '/Matrix Concatenate'], 'ConcatenateDimension', num2str(1));
      |     
      |     % Add wire to output
      |     add_line(gcb, 'Matrix Concatenate/1', 'Vector/1');
      | 
      |     % Add slice blocks and connect wires
      |     for i = 0:N-1
      |         add_block('hdlsllib/Logic and Bit Operations/Bit Slice',...
      |             [gcb, '/Bit Slice', num2str(i)],...
      |             'Position', [0 82+i*90 45 128+i*90]);
      |         set_param([gcb, '/Bit Slice', num2str(i)], 'ridx', num2str(0+i*(w)));
      |         set_param([gcb, '/Bit Slice', num2str(i)], 'lidx', num2str((w-1)+i*(w)));
      |         add_line(gcb, 'SSR/1', ['Bit Slice', num2str(i), '/1'],...
      |             'autorouting', 'on');
      |         add_line(gcb, ['Bit Slice', num2str(i), '/1'],...
      |             ['Matrix Concatenate/', num2str(i+1)],...
      |             'autorouting', 'on');
      |     end
      |     
      |     % Set the hidden attribute to prevent unnecessary changes in
      |     % architecture while generating HDL Code.
      |     set_param(gcb, 'hN', get_param(gcb, 'N'));
      |     set_param(gcb, 'hw', get_param(gcb, 'w'));
      | end
      mask DialogControl DescGroupVar Prompt: SSR to Vector
      mask DialogControl DescTextVar Prompt: Convert the SSR vector format based on the wordlength and expected number of samples per clock cycle.
  Terminator : Terminator
  Data Out : Outport
  wires:
  Data/1 -> SSR to Vector Low/1(SSR)
  Bit Slice Imag1/1 -> Real-Imag to Complex1/2
  Bit Slice Real1/1 -> Real-Imag to Complex1/1
  SSR to Vector Low/1(Vector) -> Bit Slice Imag1/1, Bit Slice Real1/1
  Data Type Conversion/1 -> Data Out/1
  Valid/1 -> Terminator/1
  Real-Imag to Complex1/1 -> Data Type Conversion/1

== system gm_spectrum_analyser/Stimulus and Channel/Transmitter/Transmitter/Vector to SSR Low ==
  Vector : Inport
  Bit Concat : hdlsllib/Logic and Bit Operations/Bit Concat  numInputs=4
  Selector0 : Selector  InputPortWidth=4  IndexOptions=Index vector (dialog)  Indices=4  OutputSizes=1
  Selector1 : Selector  InputPortWidth=4  IndexOptions=Index vector (dialog)  Indices=3  OutputSizes=1
  Selector2 : Selector  InputPortWidth=4  IndexOptions=Index vector (dialog)  Indices=2  OutputSizes=1
  Selector3 : Selector  InputPortWidth=4  IndexOptions=Index vector (dialog)  Indices=1  OutputSizes=1
  SSR : Outport
  wires:
  Bit Concat/1 -> SSR/1
  Vector/1 -> Selector0/1, Selector1/1, Selector2/1, Selector3/1
  Selector0/1 -> Bit Concat/1
  Selector1/1 -> Bit Concat/2
  Selector2/1 -> Bit Concat/3
  Selector3/1 -> Bit Concat/4

== system gm_spectrum_analyser/DDR Memory/AXI Read Interface Response Model/DDR/Enabled Subsystem/latch ==
  e : Inport  OutDataTypeStr=boolean
  d : Inport  Port=2
  Switch : Switch  Criteria=u2 > Threshold
  Unit Delay : UnitDelay  SampleTime=-1  HasFrameUpgradeWarning=on
  q : Outport  VectorParamsAs1DForOutWhenUnconnected=off
  wires:
  Switch/1 -> Unit Delay/1, q/1
  e/1 -> Switch/2
  Unit Delay/1 -> Switch/3
  d/1 -> Switch/1

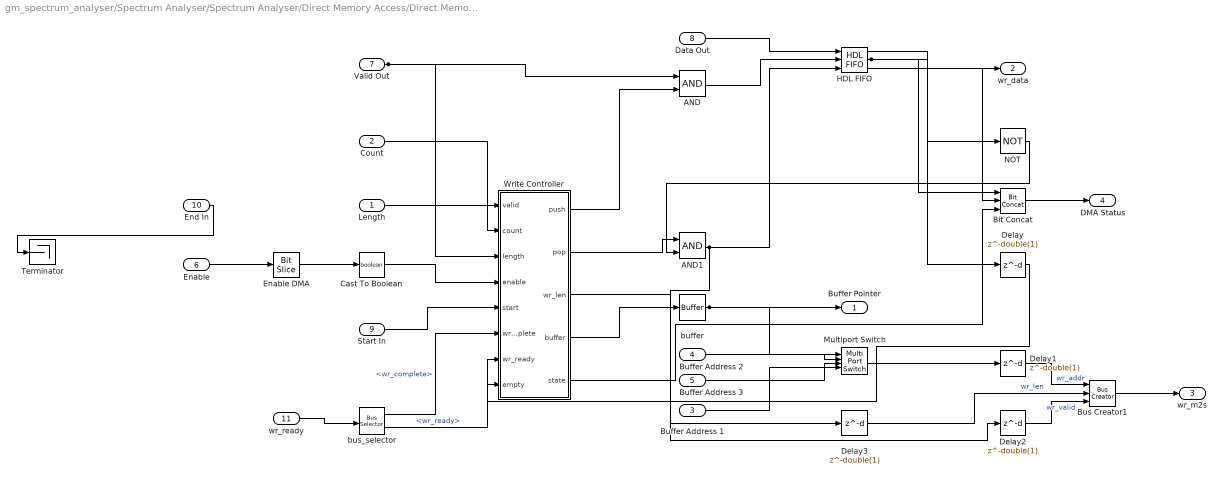
== system gm_spectrum_analyser/Spectrum Analyser/Spectrum Analyser/Direct Memory Access/Direct Memory Access/DDR Communication ==
  Length : Inport  OutDataTypeStr=uint32  PortDimensions=1  SampleTime=3.90625e-09
  Count : Inport  Port=2  OutDataTypeStr=uint32  PortDimensions=1  SampleTime=3.90625e-09
  Buffer Address 1 : Inport  Port=3  OutDataTypeStr=uint32  PortDimensions=1  SampleTime=3.90625e-09
  Buffer Address 2 : Inport  Port=4  OutDataTypeStr=uint32  PortDimensions=1  SampleTime=3.90625e-09
  Buffer Address 3 : Inport  Port=5  OutDataTypeStr=uint32  PortDimensions=1  SampleTime=3.90625e-09
  Enable : Inport  Port=6  OutDataTypeStr=uint32  PortDimensions=1  SampleTime=3.90625e-09
  Valid Out : Inport  Port=7  OutDataTypeStr=boolean  PortDimensions=1  SampleTime=3.90625e-09
  Data Out : Inport  Port=8  OutDataTypeStr=uint32  PortDimensions=1  SampleTime=3.90625e-09
  Start In : Inport  Port=9  OutDataTypeStr=boolean  PortDimensions=1  SampleTime=3.90625e-09
  End In : Inport  Port=10  OutDataTypeStr=boolean  PortDimensions=1  SampleTime=3.90625e-09
  wr_ready : Inport  Port=11  SampleTime=3.90625e-09
  AND : Logic  AllPortsSameDT=off  OutDataTypeStr=boolean  SampleTime=3.90625e-09
  AND1 : Logic  AllPortsSameDT=off  OutDataTypeStr=boolean  SampleTime=3.90625e-09
  Bit Concat : hdlsllib/Logic and Bit Operations/Bit Concat  numInputs=3
  Bus Creator1 : BusCreator  Inputs=3
  Cast To Boolean : DataTypeConversion  OutDataTypeStr=boolean  SampleTime=3.90625e-09
  Delay{,1..3} (4 alike) : Delay  DelayLength=double(1)  InitialCondition=0  SampleTime=3.90625e-09
  Enable DMA : hdlsllib/Logic and Bit Operations/Bit Slice  lidx=double(0)  ridx=double(0)
      settings: SourceProductBaseCode=SL
  HDL FIFO : hdlsllib/HDL RAMs/HDL FIFO  fifo_size=8192  mode=Classic  ratio=1  push_msg=Error  pop_msg=Error  show_empty=on  show_full=on  show_num=off  LabelModeActiveChoice_Mode=Classic
      settings: SourceProductBaseCode=SL
  Multiport Switch : MultiPortSwitch  DataPortOrder=Zero-based contiguous  DiagnosticForDefault=None  zeroidx=on  OutDataTypeStr=uint32  SampleTime=3.90625e-09
  NOT : Logic  Operator=NOT  Inputs=1  AllPortsSameDT=off  OutDataTypeStr=boolean  SampleTime=3.90625e-09
  Terminator : Terminator
  Write Controller : Subsystem
  buffer : hdlmdlgenlib/Buffer
      settings: SourceProductBaseCode=SL
  bus_selector : BusSelector  OutputSignals=wr_complete,wr_ready
  Buffer Pointer : Outport
  wr_data : Outport  Port=2
  wr_m2s : Outport  Port=3  VectorParamsAs1DForOutWhenUnconnected=off
  DMA Status : Outport  Port=4
  wires:
  Bit Concat/1 -> DMA Status/1
  Bus Creator1/1 -> wr_m2s/1
  bus_selector/1 -> Write Controller/6(wr_complete)  "<wr_complete>"
  bus_selector/2 -> Write Controller/7(wr_ready)  "<wr_ready>"
  Cast To Boolean/1 -> Write Controller/4(enable)
  Delay1/1 -> Bus Creator1/1  "wr_addr"
  Delay2/1 -> Bus Creator1/3  "wr_valid"
  Delay3/1 -> Bus Creator1/2  "wr_len"
  Enable DMA/1 -> Cast To Boolean/1
  Multiport Switch/1 -> Delay1/1
  buffer/1 -> Multiport Switch/1, Buffer Pointer/1
  AND1/1 -> Delay2/1, HDL FIFO/3
  HDL FIFO/1 -> wr_data/1
  HDL FIFO/2 -> Bit Concat/1, NOT/1, Delay/1
  HDL FIFO/3 -> Bit Concat/2
  Write Controller/3(wr_len) -> Delay3/1
  Write Controller/4(buffer) -> buffer/1
  Write Controller/5(state) -> Bit Concat/3
  Length/1 -> Write Controller/3(length)
  Count/1 -> Write Controller/2(count)
  Buffer Address 1/1 -> Multiport Switch/4
  Buffer Address 2/1 -> Multiport Switch/2
  Buffer Address 3/1 -> Multiport Switch/3
  Enable/1 -> Enable DMA/1
  Valid Out/1 -> AND/1, Write Controller/1(valid)
  Data Out/1 -> HDL FIFO/1
  Start In/1 -> Write Controller/5(start)
  End In/1 -> Terminator/1
  wr_ready/1 -> bus_selector/1
  NOT/1 -> AND1/2
  AND/1 -> HDL FIFO/2
  Delay/1 -> Write Controller/8(empty)
  Write Controller/1(push) -> AND/2
  Write Controller/2(pop) -> AND1/1

== system gm_spectrum_analyser/Spectrum Analyser/Spectrum Analyser/Spectrum Analyser Core/FFT and Spectrum Processing/Convert Data ==
  Valid Real : Inport  OutDataTypeStr=boolean  PortDimensions=1  SampleTime=3.90625e-09
  Valid Imag : Inport  Port=2  OutDataTypeStr=boolean  PortDimensions=1  SampleTime=3.90625e-09
  Data Real : Inport  Port=3  OutDataTypeStr=uint16  PortDimensions=1  SampleTime=3.90625e-09
  Data Imag : Inport  Port=4  OutDataTypeStr=uint16  PortDimensions=1  SampleTime=3.90625e-09
  AND : Logic  AllPortsSameDT=off  OutDataTypeStr=boolean  SampleTime=3.90625e-09
  Data Type Conversion : DataTypeConversion  OutDataTypeStr=fixdt(1, 16, 15)  ConvertRealWorld=Stored Integer (SI)  SampleTime=3.90625e-09
  Data Type Conversion1 : DataTypeConversion  OutDataTypeStr=fixdt(1, 16, 15)  ConvertRealWorld=Stored Integer (SI)  SampleTime=3.90625e-09
  Real-Imag to Complex : RealImagToComplex  ConstantPart="fi(0,1,16,15,\"hex\",\"0000\")"  SampleTime=3.90625e-09
  Data Out : Outport
  Valid : Outport  Port=2
  wires:
  AND/1 -> Valid/1
  Data Type Conversion/1 -> Real-Imag to Complex/1
  Data Type Conversion1/1 -> Real-Imag to Complex/2
  Real-Imag to Complex/1 -> Data Out/1
  Valid Real/1 -> AND/1
  Valid Imag/1 -> AND/2
  Data Real/1 -> Data Type Conversion/1
  Data Imag/1 -> Data Type Conversion1/1
